simulink model "Controllo_Robusto"  (R2023a)
settings: Solver=VariableStepAuto  StartTime=0.0  StopTime=113  RelTol=1e-3
values from neighbouring files (symbols this model uses):
  a1 = 0.5    [Progetto_FoR.m]
  d0 = 1    [Progetto_FoR.m]
  KD = diag(kd)    [Progetto_FoR.m]
  KD2 = diag(kd2)    [Progetto_FoR.m]
  KP = diag(kp)    [Progetto_FoR.m]
  KP2 = diag(kp2)    [Progetto_FoR.m]
  pi0 = [ml1 Il1 Im1 Fm1 ml2 Il2 Im2 Fm2 ml3 Im3 Fm3 Il4 Im4 Fm4]    [Progetto_FoR.m]
  q0 = [0 pi/2 0 pi/2]    [Progetto_FoR.m]
  Tc = 0.001    [Progetto_FoR.m]
undefined symbols (not defined in the file or in its folder): DiscIntNeverNeededParam
settings Model: Creator=panto  LastModifiedBy=panto

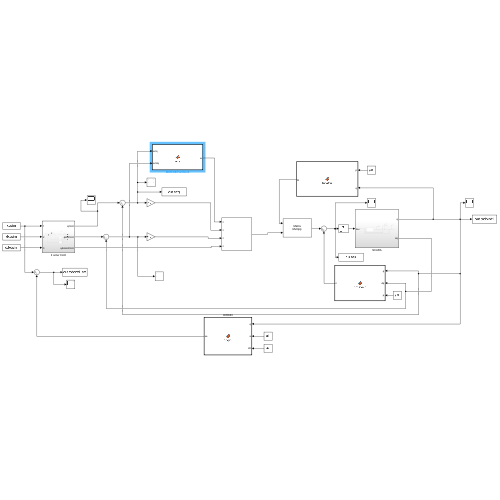
[thumbnail: Simulink's stored preview of the top-level diagram]
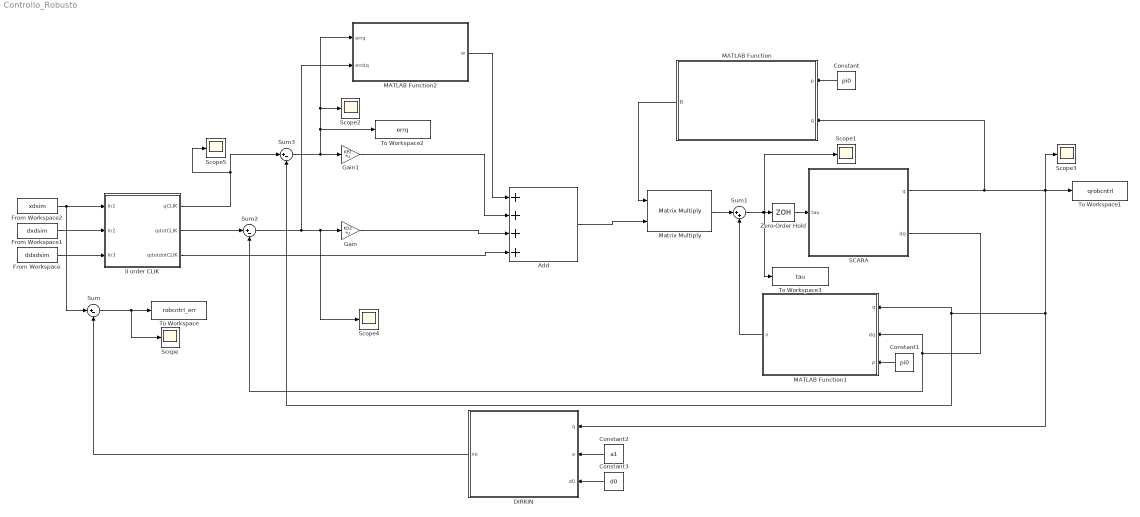
== system Controllo_Robusto ==
  Add : Sum  Inputs=++++
  Constant : Constant  Value=pi0
  Constant1 : Constant  Value=pi0
  Constant2 : Constant  Value=a1
  Constant3 : Constant  Value=d0
  DIRKIN : MATLAB Function  TreatAsAtomicUnit=on
  From Workspace : FromWorkspace  VariableName=ddxdsim  SampleTime=Tc
  From Workspace1 : FromWorkspace  VariableName=dxdsim  SampleTime=Tc
  From Workspace2 : FromWorkspace  VariableName=xdsim  SampleTime=Tc
  Gain : Gain  Gain=KD2  Multiplication=Matrix(K*u)
  Gain1 : Gain  Gain=KP2  Multiplication=Matrix(K*u)
  II order CLIK : Subsystem
  MATLAB Function : MATLAB Function  TreatAsAtomicUnit=on
  MATLAB Function1 : MATLAB Function  TreatAsAtomicUnit=on
  MATLAB Function2 : MATLAB Function  TreatAsAtomicUnit=on
  Matrix Multiply : Product  Multiplication=Matrix(*)
  SCARA : Subsystem
  Scope{,1..5} (6 alike) : Scope
  Sum : Sum  Inputs=|+-
  Sum1 : Sum  Inputs=|++
  Sum2 : Sum  Inputs=|+-
  Sum3 : Sum  Inputs=|+-
  To Workspace : ToWorkspace  VariableName=robcntrl_err  SampleTime=Tc
      settings: Save2DSignal=2-D array (concatenate along first dimension)
  To Workspace1 : ToWorkspace  VariableName=qrobcntrl  SampleTime=-1
      settings: Save2DSignal=2-D array (concatenate along first dimension)
  To Workspace2 : ToWorkspace  VariableName=errq  SampleTime=-1
      settings: Save2DSignal=2-D array (concatenate along first dimension)
  To Workspace3 : ToWorkspace  VariableName=tau  SampleTime=-1
      settings: Save2DSignal=2-D array (concatenate along first dimension)
  Zero-Order Hold : ZeroOrderHold  SampleTime=-1
  wires:
  From Workspace2/1 -> II order CLIK/1(In1), Sum/1
  From Workspace1/1 -> II order CLIK/2(In2)
  From Workspace/1 -> II order CLIK/3(In3)
  Constant3/1 -> DIRKIN/3(d0)
  Constant2/1 -> DIRKIN/2(a)
  DIRKIN/1(xe) -> Sum/2
  Sum/1 -> Scope/1, To Workspace/1
  MATLAB Function/1(B) -> Matrix Multiply/1
  Matrix Multiply/1 -> Sum1/1
  Sum1/1 -> To Workspace3/1, Scope1/1, Zero-Order Hold/1
  MATLAB Function1/1(n) -> Sum1/2
  II order CLIK/1(qCLIK) -> Scope5/1, Sum3/1
  II order CLIK/3(qdotdotCLIK) -> Add/4
  II order CLIK/2(qdotCLIK) -> Sum2/1
  Sum2/1 -> MATLAB Function2/2(errdq), Scope4/1, Gain/1
  Sum3/1 -> To Workspace2/1, Scope2/1, MATLAB Function2/1(errq), Gain1/1
  MATLAB Function2/1(w) -> Add/1
  Gain/1 -> Add/3
  Gain1/1 -> Add/2
  Add/1 -> Matrix Multiply/2
  SCARA/1(q) -> MATLAB Function/2(q), DIRKIN/1(q), MATLAB Function1/1(q), Sum3/2, Scope3/1, To Workspace1/1
  SCARA/2(dq) -> MATLAB Function1/2(dq), Sum2/2
  Zero-Order Hold/1 -> SCARA/1(tau)
  Constant/1 -> MATLAB Function/1(p)
  Constant1/1 -> MATLAB Function1/3(p)

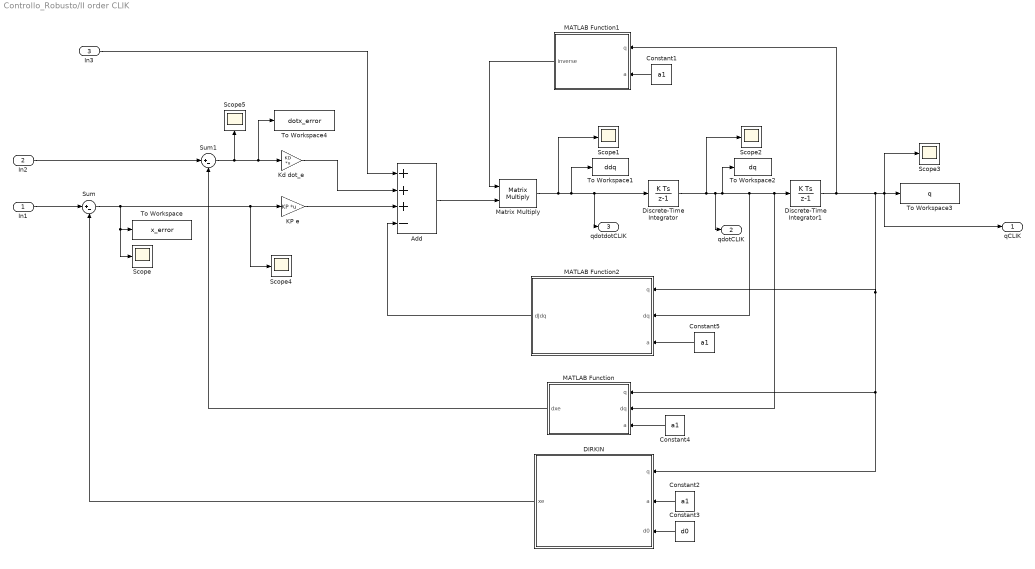
== system Controllo_Robusto/II order CLIK ==
  In1 : Inport
  In2 : Inport  Port=2
  In3 : Inport  Port=3
  Add : Sum  Inputs=+++-
  Constant{1..2,4..5} (4 alike) : Constant  Value=a1
  Constant3 : Constant  Value=d0
  DIRKIN : MATLAB Function  TreatAsAtomicUnit=on
  Discrete-Time Integrator : DiscreteIntegrator  InitialCondition=[0;0;0;0]  SampleTime=Tc  ICPrevOutput=DiscIntNeverNeededParam  ICPrevScaledInput=DiscIntNeverNeededParam
  Discrete-Time Integrator1 : DiscreteIntegrator  InitialCondition=q0'  SampleTime=Tc  ICPrevOutput=DiscIntNeverNeededParam  ICPrevScaledInput=DiscIntNeverNeededParam
  KP e : Gain  Gain=KP  Multiplication=Matrix(K*u)
  Kd dot_e : Gain  Gain=KD  Multiplication=Matrix(K*u)
  MATLAB Function : MATLAB Function  TreatAsAtomicUnit=on
  MATLAB Function1 : MATLAB Function  TreatAsAtomicUnit=on
  MATLAB Function2 : MATLAB Function  TreatAsAtomicUnit=on
  Matrix Multiply : Product  Multiplication=Matrix(*)
  Scope{,1..5} (6 alike) : Scope
  Sum : Sum  Inputs=|+-
  Sum1 : Sum  Inputs=|+-
  To Workspace : ToWorkspace  VariableName=x_error  SampleTime=Tc
      settings: Save2DSignal=2-D array (concatenate along first dimension)
  To Workspace1 : ToWorkspace  VariableName=ddq  SampleTime=-1
      settings: Save2DSignal=2-D array (concatenate along first dimension)
  To Workspace2 : ToWorkspace  VariableName=dq  SampleTime=-1
      settings: Save2DSignal=2-D array (concatenate along first dimension)
  To Workspace3 : ToWorkspace  VariableName=q  SampleTime=Tc
      settings: Save2DSignal=2-D array (concatenate along first dimension)
  To Workspace4 : ToWorkspace  VariableName=dotx_error  SampleTime=-1
      settings: Save2DSignal=2-D array (concatenate along first dimension)
  qCLIK : Outport
  qdotCLIK : Outport  Port=2
  qdotdotCLIK : Outport  Port=3
  wires:
  Discrete-Time Integrator/1 -> Scope2/1, qdotCLIK/1, To Workspace2/1, MATLAB Function2/2(dq), MATLAB Function/2(dq), Discrete-Time Integrator1/1
  Sum/1 -> Scope/1, To Workspace/1, Scope4/1, KP e/1
  Kd dot_e/1 -> Add/2
  In2/1 -> Sum1/1
  Constant5/1 -> MATLAB Function2/3(a)
  Constant1/1 -> MATLAB Function1/2(a)
  Constant3/1 -> DIRKIN/3(d0)
  KP e/1 -> Add/3
  Matrix Multiply/1 -> Scope1/1, To Workspace1/1, qdotdotCLIK/1, Discrete-Time Integrator/1
  MATLAB Function/1(dxe) -> Sum1/2
  Constant4/1 -> MATLAB Function/3(a)
  Add/1 -> Matrix Multiply/2
  In3/1 -> Add/1
  Discrete-Time Integrator1/1 -> MATLAB Function2/1(q), MATLAB Function/1(q), DIRKIN/1(q), Scope3/1, qCLIK/1, To Workspace3/1, MATLAB Function1/1(q)
  In1/1 -> Sum/1
  MATLAB Function2/1(dJdq) -> Add/4
  DIRKIN/1(xe) -> Sum/2
  Constant2/1 -> DIRKIN/2(a)
  MATLAB Function1/1(inverse) -> Matrix Multiply/1
  Sum1/1 -> Scope5/1, To Workspace4/1, Kd dot_e/1

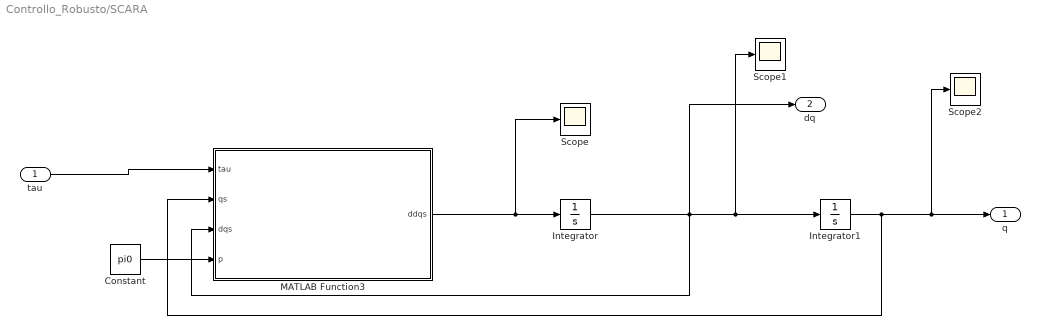
== system Controllo_Robusto/SCARA ==
  tau : Inport
  Constant : Constant  Value=pi0
  Integrator : Integrator  InitialCondition=[0;0;0;0]
  Integrator1 : Integrator  InitialCondition=q0'
  MATLAB Function3 : MATLAB Function  TreatAsAtomicUnit=on
  Scope : Scope
  Scope1 : Scope
  Scope2 : Scope
  q : Outport  SampleTime=Tc
  dq : Outport  Port=2  SampleTime=Tc
  wires:
  Integrator/1 -> dq/1, MATLAB Function3/3(dqs), Integrator1/1, Scope1/1
  tau/1 -> MATLAB Function3/1(tau)
  Integrator1/1 -> MATLAB Function3/2(qs), Scope2/1, q/1
  MATLAB Function3/1(ddqs) -> Integrator/1, Scope/1
  Constant/1 -> MATLAB Function3/4(p)

== matlab function Controllo_Robusto/II order CLIK/MATLAB Function1 ==
  data: q input; inverse output; a input
function inverse = invJ(q,a)
%devo prima calcolare lo Jacobiano analitico e poi invertirlo
%Nel caso dello SCARA, lo Jacobiano analitico coincide con quello
%geometrico: questo perchè nello SCARA l'orientamento può essere
%rappresentato direttamente dall'angolo attorno a z, e quindi la velocità
%angolare z si traduce direttamente nella velocità di cambiamento
%dell'angolo di orientamento attorno z
%dal libro when the DOFs cause rotations of the end-effector all about the 
% same fixed axis in space, the two Jacobians are essentially the same
   
    Ja = zeros(4,4);
    Ja = [-a*sin(q(1)+q(2))-a*sin(q(1)) -a*sin(q(1)+q(2)) 0 0;
        a*cos(q(1)+q(2))+a*cos(q(1)) a*cos(q(1)+q(2)) 0 0;
        0 0 -1 0;
        1 1 0 -1];

    inverse = inv(Ja);

end

== matlab function Controllo_Robusto/II order CLIK/DIRKIN ==
  data: q input; xe output; a input; d0 input
function xe = dirkyn(q, a, d0)
  xe = zeros(4,1);
    xe = [a*cos(q(1)+q(2))+a*cos(q(1));
        a*sin(q(1)+q(2))+a*sin(q(1));
        d0-q(3);
        q(1)+q(2)-q(4)];
end

== matlab function Controllo_Robusto/II order CLIK/MATLAB Function ==
  data: q input; dq input; dxe output; a input
function dxe = Ja(q,dq,a)

Ja = zeros(4,4);
Ja = [-a*sin(q(1)+q(2))-a*sin(q(1)) -a*sin(q(1)+q(2)) 0 0;
        a*cos(q(1)+q(2))+a*cos(q(1)) a*cos(q(1)+q(2)) 0 0;
        0 0 -1 0;
        1 1 0 -1];

    dxe = Ja*dq;

end

== matlab function Controllo_Robusto/II order CLIK/MATLAB Function2 ==
  data: q input; dq input; dJdq output; a input
function dJdq =  dotJadotq(q,dq,a)
    
    dotJa = zeros(4,4);
    dotJa = [-a*cos(q(1))*dq(1)-a*cos(q(1)+q(2))*(dq(1)+dq(2)) -a*cos(q(1)+q(2))*(dq(1)+dq(2)) 0 0;
        -a*sin(q(1))*dq(1)-a*sin(q(1)+q(2))*(dq(1)+dq(2)) -a*sin(q(1)+q(2))*(dq(1)+dq(2)) 0 0;
        0 0 0 0;
        0 0 0 0];

    dJdq = dotJa*dq;

end

== matlab function Controllo_Robusto/DIRKIN ==
  data: q input; xe output; a input; d0 input
function xe = dirkyn(q, a, d0)
  xe = zeros(4,1);
    xe = [a*cos(q(1)+q(2))+a*cos(q(1));
        a*sin(q(1)+q(2))+a*sin(q(1));
        d0-q(3);
        q(1)+q(2)-q(4)];
end

== matlab function Controllo_Robusto/MATLAB Function ==
  data: p input; q input; B output
function B = Bmatrix(p, q)
%funzioni per il calcolo della matrice di inerzia
%I valori numerici sono i valori delle costanti del modello
    mp = 0; %Payload
    b11 = p(2)+p(6)+p(12)+p(1)*0.0625+p(5)*(0.25+0.0625+0.25*cos(q(2))) + p(9)*(0.5+0.5*cos(q(2)))+p(3);
    b22 = p(6) + p(12) + p(5)*0.0625 + p(9)*0.25 + p(7);
    b33 = p(9) +2500*p(10);
    b44 = p(12) + 400*p(13);
    b12 = p(2) + p(12) + p(5)*(0.0625+0.125*cos(q(2))) + p(9)*(0.25+0.25*cos(q(2)));
    b21 = b12;
    b14 = -p(12);
    b41 = b14;
    b24 = b14;
    b42 = b14;
    
    B = [b11 b12 0 b14;
        b21 b22 0 b24;
        0 0 b33 0;
        b41 b42 0 b44];

end

== matlab function Controllo_Robusto/MATLAB Function1 ==
  data: q input; n output; dq input; p input
function n = nonlinear(q,dq,p)

mp = 0;  %massa di un eventuale carico in punta
k = -p(5)*0.125*sin(q(2)) - (p(9)+mp)*0.25*sin(q(2)); %costante per la matrice C
gr = 9.81;
g = [0; 0; -gr*(p(9)+mp); 0];

%Matrice degli attriti viscosi
f_v = [p(4) p(8) 2500*p(11) 400*p(14)];
F_v = diag(f_v);

C = [k*dq(2) k*(dq(1)+dq(2)) 0 0;
    -k*dq(1) 0 0 0;
    0 0 0 0;
    0 0 0 0];

n = C*dq +g;
%C*dq +F_v*dq, non modello l'attrito, è questa l'imperfezione
end

== matlab function Controllo_Robusto/MATLAB Function2 ==
  data: errq input; w output; errdq input
function w = vers(errq,errdq)

rho = 70;
eps = 0.01;
xi = [errq;errdq];
O = zeros(4,4);
I = eye(4);
D = [O;I];
q1 = [200 200 200 200];
q2 = [0.1 0.1 0.1 0.1];
Q1 = diag(q1);
Q2 = diag(q2);
Q = [Q1 Q1;
    Q1 Q2];

z = D'*Q*xi;

if norm(z) >= eps
    w = (rho*z)/norm(z);
else
    w = (rho*z)/eps;
end

end

== matlab function Controllo_Robusto/SCARA/MATLAB Function3 ==
  data: tau input; ddqs output; qs input; dqs input; p input
function ddqs = SCARA(tau,qs,dqs,p)
    %devo implementare l'equazione ddq = B^-1 (tau-tau')
    %inizio calcolando B
    b11 = p(2)+p(6)+p(12)+p(1)*0.0625+p(5)*(0.25+0.0625+0.25*cos(qs(2))) + p(9)*(0.5+0.5*cos(qs(2)))+p(3);
    b22 = p(6) + p(12) + p(5)*0.0625 + p(9)*0.25 + p(7);
    b33 = p(9) +2500*p(10);
    b44 = p(12) + 400*p(13);
    b12 = p(2) + p(12) + p(5)*(0.0625+0.125*cos(qs(2))) + p(9)*(0.25+0.25*cos(qs(2)));
    b21 = b12;
    b14 = -p(12);
    b41 = b14;
    b24 = b14;
    b42 = b14;
    
    B = [b11 b12 0 b14;
        b21 b22 0 b24;
        0 0 b33 0;
        b41 b42 0 b44];
    %poi mi servono C, Fv e gravità

    k = -p(5)*0.125*sin(qs(2)) - p(9)*0.25*sin(qs(2)); %costante per la matrice C
    gr = 9.81;
    mp = 3; %Payload
    g = [0; 0; -gr*(p(9)+mp); 0];

    %Matrice degli attriti viscosi
    f_v = [0.00005 0.00005 25 2];
    F_v = diag(f_v);

    C = [k*dqs(2) k*(dqs(1)+dqs(2)) 0 0;
         -k*dqs(1) 0 0 0;
            0 0 0 0;
            0 0 0 0];
    
    tau_primo = C*dqs+F_v*dqs +g;
   
    ddqs = inv(B)*(tau-tau_primo);


end
